simulink model "Model"  (R2021a)
settings: Solver=VariableStepAuto  StartTime=0.0  StopTime=15000  RelTol=1e-3
settings Model: Creator=alaba  LastModifiedBy=alaba

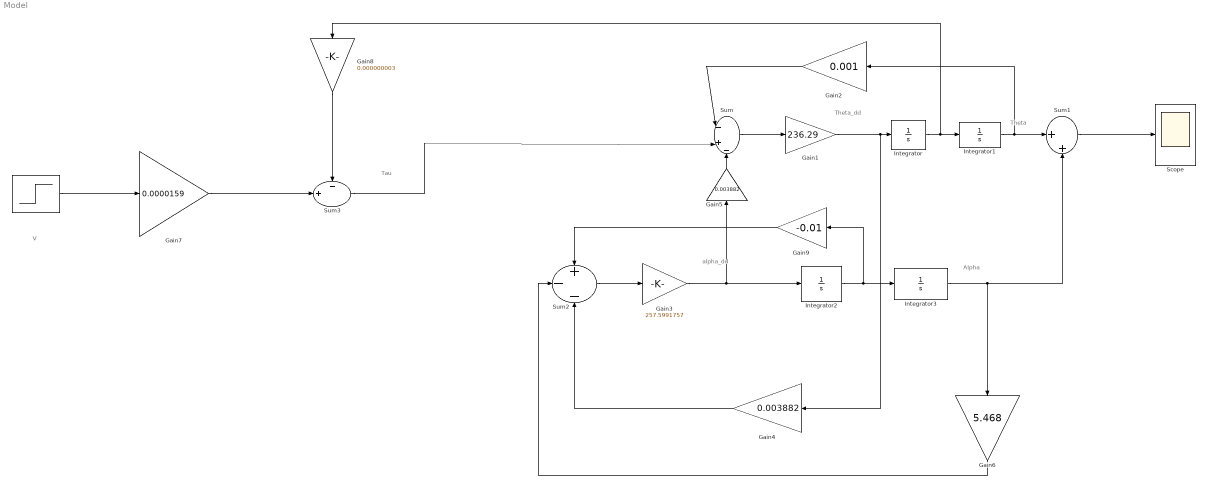
== system Model ==
  note: Theta
  note: Alpha
  note: alpha_dd
  note: Theta_dd
  note: Tau
  note: V
  " " : Step  After=5  SampleTime=0
  Gain1 : Gain  Gain=236.29
  Gain2 : Gain  Gain=0.001
  Gain3 : Gain  Gain=257.5991757
  Gain4 : Gain  Gain=0.003882
  Gain5 : Gain  Gain=0.003882
  Gain6 : Gain  Gain=5.468
  Gain7 : Gain  Gain=0.0000159
  Gain8 : Gain  Gain=0.000000003
  Gain9 : Gain  Gain=-0.01
  Integrator{,1..3} (4 alike) : Integrator
  Scope : Scope
  Sum : Sum  Inputs=|-+-
  Sum1 : Sum  Inputs=|++
  Sum2 : Sum  Inputs=+--
  Sum3 : Sum  Inputs=-+|
  wires:
  Integrator/1 -> Integrator1/1, Gain8/1
  Integrator2/1 -> Gain9/1, Integrator3/1
  Sum/1 -> Gain1/1
  Gain1/1 -> Gain4/1, Integrator/1
  Integrator3/1 -> Sum1/2, Gain6/1
  Integrator1/1 -> Sum1/1, Gain2/1
  Gain3/1 -> Integrator2/1, Gain5/1
  Sum2/1 -> Gain3/1
  Gain5/1 -> Sum/3
  Gain7/1 -> Sum3/2
  Gain8/1 -> Sum3/1
  Sum3/1 -> Sum/2
  Gain2/1 -> Sum/1
  Gain4/1 -> Sum2/3
  Gain6/1 -> Sum2/2
  Gain9/1 -> Sum2/1
  Sum1/1 -> Scope/1
  " "/1 -> Gain7/1
